simulink model "Lab4"  (R2020b)
settings: Solver=VariableStepAuto  StartTime=0.0  StopTime=10.0  RelTol=1e-3
settings Model: Creator=MY lenovo  LastModifiedBy=MY lenovo

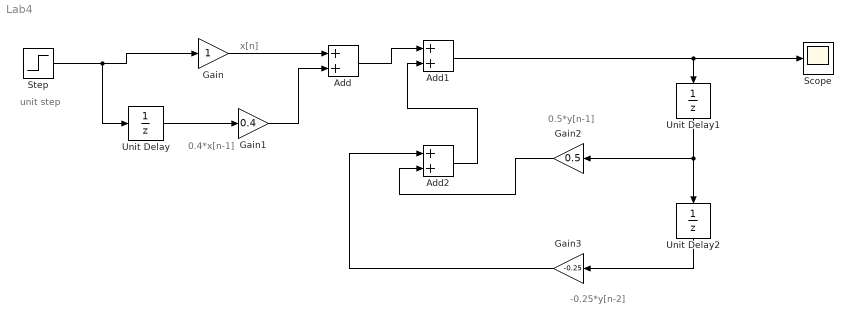
== system Lab4 ==
  note: -0.25*y[n-2]
  note: 0.5*y[n-1]
  note: 0.4*x[n-1]
  note: x[n]
  note: unit step
  Add : Sum
  Add1 : Sum
  Add2 : Sum
  Gain : Gain
  Gain1 : Gain  Gain=0.4
  Gain2 : Gain  Gain=0.5
  Gain3 : Gain  Gain=-0.25
  Scope : Scope
  Step : Step  SampleTime=0
  Unit Delay : UnitDelay  SampleTime=-1  HasFrameUpgradeWarning=on
  Unit Delay1 : UnitDelay  SampleTime=-1  HasFrameUpgradeWarning=on
  Unit Delay2 : UnitDelay  SampleTime=-1  HasFrameUpgradeWarning=on
  wires:
  Unit Delay/1 -> Gain1/1
  Gain1/1 -> Add/2
  Gain/1 -> Add/1
  Add/1 -> Add1/1
  Add2/1 -> Add1/2
  Unit Delay2/1 -> Gain3/1
  Unit Delay1/1 -> Gain2/1, Unit Delay2/1
  Gain3/1 -> Add2/1
  Gain2/1 -> Add2/2
  Step/1 -> Unit Delay/1, Gain/1
  Add1/1 -> Unit Delay1/1, Scope/1
